simulink model "real_time_optimal_control"  (R2020b)
settings: Solver=ode4  StartTime=0.0  StopTime=30  FixedStep=h_plant  RelTol=1e-3
values from neighbouring files (symbols this model uses):
  A = [zeros(3) eye(3)   zeros(3) ... (first row only)    [run_drone_estimate.m]    (also in run_simulation.m = [0 1; 0 0])
  B = [zeros(3) zeros(3) ... (first row only)    [run_drone_estimate.m]    (also in run_simulation.m = [0; 1])
  C = [eye(3) zeros(3) zeros(3)]    [run_drone_estimate.m]    (also in run_simulation.m = [1 0])
  C_discrete = [1 0]    [run_simulation.m]
  D_discrete = zeros(3,6)    [run_drone_estimate.m]    (also in run_simulation.m = 0)
  G = [zeros(3) zeros(3) ... (first row only)    [run_drone_estimate.m]
  Gamma = [h^2/2; h]    [run_simulation.m]
  h = 0.1    [run_drone_estimate.m]    (also in run_simulation.m = 1)
  h_plant = (1e-3)    (= 0.001)    [run_drone_estimate.m]    (also in run_simulation.m)
  N = 20    [run_simulation.m]
  n = length(A)    [run_drone_estimate.m]    (also in run_simulation.m = length(Phi))
  Phi = [1 h; 0 1]    [run_simulation.m]
  Q = .1*eye(2*3)    [run_drone_estimate.m]
  Q0 = eye(n)    [run_simulation.m]
  Q1 = eye(n)    [run_simulation.m]
  Q2 = 1    [run_simulation.m]
  R = .1*eye(3)    [run_drone_estimate.m]
  reference = [am;g]    [run_drone_estimate.m]    (also in run_simulation.m = 0)
  sat_max = (10000)    (= 10000)    [run_drone_estimate.m]    (also in run_simulation.m = 10)
  sat_min = -(10000)    (= -10000)    [run_drone_estimate.m]    (also in run_simulation.m = -10)
  wind_final_value = 0    [run_drone_estimate.m]    (also in run_simulation.m)
  wind_initial_value = 0    [run_drone_estimate.m]    (also in run_simulation.m)
  wind_steptime = 5    [run_drone_estimate.m]    (also in run_simulation.m)
  x0 = zeros(n, 1)    [run_drone_estimate.m]    (also in run_simulation.m = zeros(2, 1))
undefined symbols (not defined in the file or in its folder): DiscIntNeverNeededParam, Discrete, K, K_non_optimal, Time
libraries: eeLuenbergerObserver x4, simulink x1, ctrlSharedLib x1
settings Model: Creator=Trevor  LastModifiedBy=lucas
settings SolverCC: AlgebraicLoopSolver=LineSearch  AutoInsertRateTranBlk=on
settings DataIOCC: LimitDataPoints=on  SaveFormat=Array
settings OptimizationCC: LifeSpan=inf
settings DebuggingCC: SFUnexpectedBacktrackingDiag=warning  SFNoUnconditionalDefaultTransitionDiag=warning  SFExecutionAtInitializationDiag=none  UnderSpecifiedDimensionMsg=warning  ArithmeticOperatorsInVariantConditions=warning
settings HardwareCC: ProdHWDeviceType=AMD->x86-64 (Windows64)
settings ModelReferenceCC: PropagateSignalLabelsOutOfModel=off
settings SFSimCC: SimUseLocalCustomCode=off  CustomCodeUndefinedFunction=UseInterfaceOnly
settings RTWCC: RTWUseLocalCustomCode=off
settings CodeAppCC: StateflowObjectComments=on
settings GRTTargetCC: TargetLangStandard=C89/C90 (ANSI)
settings ConfigComp: CovMetricSettings=dw  CovSaveCumulativeToWorkspaceVar=on  CovSaveSingleToWorkspaceVar=on  CovExternalEMLEnable=off

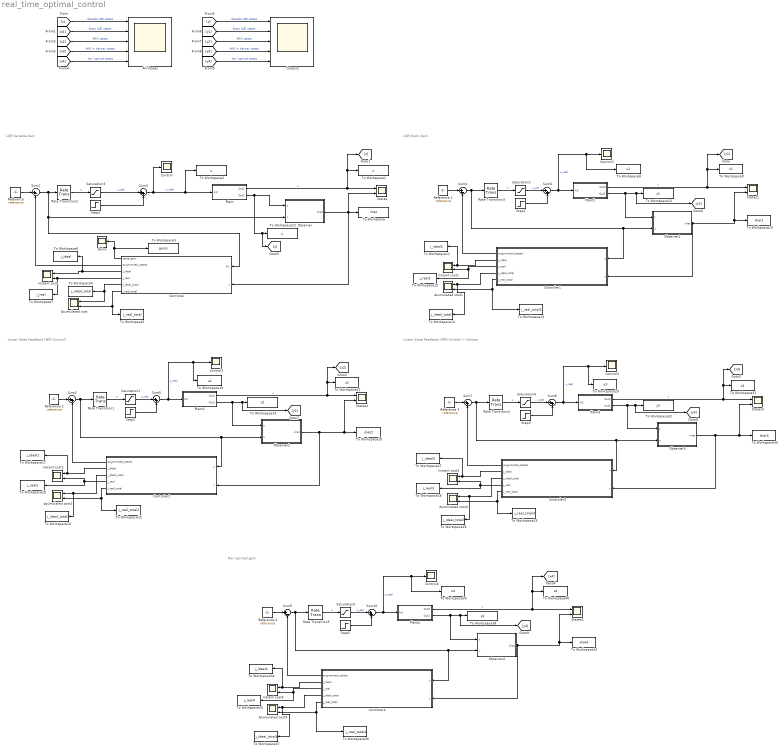
== system real_time_optimal_control ==
  note: LQR Static Gain
  note: LQR Variable Gain
  note: Linear State Feedback (MPC Control)
  note: Linear State Feedback (MPC Control) + Kalman
  note: Non optimal gain
  Acumulated cost{,1..4} (5 alike) : Scope  NumInputPorts=2
  All States : Scope  NumInputPorts=5
  Control{,1..4} (5 alike) : Scope
  Controler : Subsystem
  Controler1 : Subsystem
  Controler2 : Subsystem
  Controler3 : Subsystem
  Controler4 : Subsystem
  Gains : Scope
  Instant cost{,1..4} (5 alike) : Scope  NumInputPorts=2
  Observer : Subsystem
  Observer1 : Subsystem
  Observer2 : Subsystem
  Observer3 : Subsystem
  Observer4 : Subsystem
  Outputs : Scope  NumInputPorts=5
  Plant : Subsystem
  Plant1 : Subsystem
  Plant2 : Subsystem
  Plant3 : Subsystem
  Plant4 : Subsystem
  Rate Transition{1..5} (5 alike) : RateTransition  Integrity=off  OutPortSampleTimeMultiple=0.01  OutPortSampleTime=h_plant
  Reference : Constant  Value=reference  SampleTime=h
  Reference {1..4} (4 alike) : Constant  Value=reference  SampleTime=h
  Saturation{1..5} (5 alike) : Saturate  UpperLimit=sat_max  LowerLimit=sat_min
  States{,1..4} (5 alike) : Scope  NumInputPorts=2
  Step{1..5} (5 alike) : Step  Time=wind_steptime  Before=wind_initial_value  After=wind_final_value  SampleTime=h_plant
  Sum1 : Sum  Inputs=|+-
  Sum{2..3,5..8,10} (7 alike) : Sum  Inputs=|++
  Sum4 : Sum  Inputs=|+-
  Sum9 : Sum  Inputs=|+-
  To Workspace : ToWorkspace  VariableName=xhat  SaveFormat=Timeseries  SampleTime=-1
  To Workspace1 : ToWorkspace  VariableName=x  SaveFormat=Timeseries  SampleTime=-1
  To Workspace10 : ToWorkspace  VariableName=xhat1  SaveFormat=Timeseries  SampleTime=-1
  To Workspace11 : ToWorkspace  VariableName=j_ideal1  SaveFormat=Timeseries  SampleTime=-1
  To Workspace12 : ToWorkspace  VariableName=j_real1  SaveFormat=Timeseries  SampleTime=-1
  To Workspace13 : ToWorkspace  VariableName=j_real_total1  SaveFormat=Timeseries  SampleTime=-1
  To Workspace14 : ToWorkspace  VariableName=j_ideal_total1  SaveFormat=Timeseries  SampleTime=-1
  To Workspace15 : ToWorkspace  VariableName=j_real_total2  SaveFormat=Timeseries  SampleTime=-1
  To Workspace16 : ToWorkspace  VariableName=j_ideal_total2  SaveFormat=Timeseries  SampleTime=-1
  To Workspace17 : ToWorkspace  VariableName=j_ideal2  SaveFormat=Timeseries  SampleTime=-1
  To Workspace18 : ToWorkspace  VariableName=j_real2  SaveFormat=Timeseries  SampleTime=-1
  To Workspace19 : ToWorkspace  VariableName=u2  SaveFormat=Timeseries  SampleTime=-1
  To Workspace2 : ToWorkspace  VariableName=u  SaveFormat=Timeseries  SampleTime=-1
  To Workspace20 : ToWorkspace  VariableName=xhat2  SaveFormat=Timeseries  SampleTime=-1
  To Workspace21 : ToWorkspace  VariableName=x2  SaveFormat=Timeseries  SampleTime=-1
  To Workspace22 : ToWorkspace  VariableName=y  SaveFormat=Timeseries  SampleTime=-1
  To Workspace23 : ToWorkspace  VariableName=y1  SaveFormat=Timeseries  SampleTime=-1
  To Workspace24 : ToWorkspace  VariableName=y2  SaveFormat=Timeseries  SampleTime=-1
  To Workspace25 : ToWorkspace  VariableName=j_real_total3  SaveFormat=Timeseries  SampleTime=-1
  To Workspace26 : ToWorkspace  VariableName=j_ideal_total3  SaveFormat=Timeseries  SampleTime=-1
  To Workspace27 : ToWorkspace  VariableName=j_ideal3  SaveFormat=Timeseries  SampleTime=-1
  To Workspace28 : ToWorkspace  VariableName=j_real3  SaveFormat=Timeseries  SampleTime=-1
  To Workspace29 : ToWorkspace  VariableName=u3  SaveFormat=Timeseries  SampleTime=-1
  To Workspace3 : ToWorkspace  VariableName=gains  SaveFormat=Timeseries  SampleTime=-1
  To Workspace30 : ToWorkspace  VariableName=xhat3  SaveFormat=Timeseries  SampleTime=-1
  To Workspace31 : ToWorkspace  VariableName=x3  SaveFormat=Timeseries  SampleTime=-1
  To Workspace32 : ToWorkspace  VariableName=y3  SaveFormat=Timeseries  SampleTime=-1
  To Workspace33 : ToWorkspace  VariableName=xhat4  SaveFormat=Timeseries  SampleTime=-1
  To Workspace34 : ToWorkspace  VariableName=j_ideal4  SaveFormat=Timeseries  SampleTime=-1
  To Workspace35 : ToWorkspace  VariableName=j_real4  SaveFormat=Timeseries  SampleTime=-1
  To Workspace36 : ToWorkspace  VariableName=j_real_total4  SaveFormat=Timeseries  SampleTime=-1
  To Workspace37 : ToWorkspace  VariableName=j_ideal_total4  SaveFormat=Timeseries  SampleTime=-1
  To Workspace38 : ToWorkspace  VariableName=y4  SaveFormat=Timeseries  SampleTime=-1
  To Workspace39 : ToWorkspace  VariableName=u4  SaveFormat=Timeseries  SampleTime=-1
  To Workspace4 : ToWorkspace  VariableName=j_ideal_total  SaveFormat=Timeseries  SampleTime=-1
  To Workspace40 : ToWorkspace  VariableName=x4  SaveFormat=Timeseries  SampleTime=-1
  To Workspace5 : ToWorkspace  VariableName=j_real_total  SaveFormat=Timeseries  SampleTime=-1
  To Workspace6 : ToWorkspace  VariableName=j_ideal  SaveFormat=Timeseries  SampleTime=-1
  To Workspace7 : ToWorkspace  VariableName=j_real  SaveFormat=Timeseries  SampleTime=-1
  To Workspace8 : ToWorkspace  VariableName=u1  SaveFormat=Timeseries  SampleTime=-1
  To Workspace9 : ToWorkspace  VariableName=x1  SaveFormat=Timeseries  SampleTime=-1
  wires:
  Plant/2(Out1) -> [y], To Workspace22/1, Observer/1(y)
  Saturation3/1 -> Sum3/1  "u_sat"
  Sum3/1 -> Control/1, Plant/1(In2), To Workspace2/1  "u_real"
  Step4/1 -> Sum3/2
  Plant/1(Out2) -> [x], To Workspace1/1, States/1  "x"
  Reference/1 -> Sum1/1
  Rate Transition2/1 -> Saturation3/1  "u"
  Sum6/1 -> Plant1/1(In2), To Workspace8/1, Control1/1  "u_real"
  Step1/1 -> Sum6/2
  Plant1/1(Out2) -> [x1], To Workspace9/1, States1/1  "x"
  Reference 1/1 -> Sum4/1
  Sum4/1 -> Controler1/1(u), Observer1/2(u), Rate Transition3/1
  Observer1/1(xhat) -> Controler1/2(x), To Workspace10/1, States1/2
  Saturation1/1 -> Sum6/1  "u_sat"
  Plant1/2(Out1) -> Observer1/1(y), [y1], To Workspace23/1
  Rate Transition3/1 -> Saturation1/1  "u"
  Rate Transition1/1 -> Saturation2/1  "u"
  Saturation2/1 -> Sum5/1  "u_sat"
  Plant2/2(Out1) -> Observer2/1(y), [y2], To Workspace24/1
  Plant2/1(Out2) -> [x2], To Workspace21/1, States2/1  "x"
  Step2/1 -> Sum5/2
  Sum5/1 -> Plant2/1(In2), To Workspace19/1, Control2/1  "u_real"
  Sum2/1 -> Controler2/1(u), Observer2/2(u), Rate Transition1/1
  Reference 2/1 -> Sum2/1
  Sum1/1 -> Controler/1(In1), Observer/2(u), Rate Transition2/1
  Observer/1(xhat) -> To Workspace/1, Controler/2(x), States/2
  Controler/1(state_gain) -> To Workspace3/1, Gains/1
  Controler/2(augmented_states) -> Sum1/2
  Controler/3(j_ideal) -> To Workspace6/1, Instant cost/1
  Controler/4(j_real) -> To Workspace7/1, Instant cost/2
  Controler/5(j_ideal_total) -> Acumulated cost/1, To Workspace4/1
  Controler/6(j_real_total) -> To Workspace5/1, Acumulated cost/2
  Controler1/1(augmented_states) -> Sum4/2
  Controler1/2(j_ideal) -> To Workspace11/1, Instant cost1/1
  Controler1/3(j_real) -> To Workspace12/1, Instant cost1/2
  Controler1/4(j_ideal_total) -> To Workspace14/1, Acumulated cost1/1
  Controler1/5(j_real_total) -> To Workspace13/1, Acumulated cost1/2
  Controler2/3(j_ideal_total) -> To Workspace16/1, Acumulated cost2/1
  Controler2/5(j_real_total) -> To Workspace15/1, Acumulated cost2/2
  Controler2/2(j_ideal) -> To Workspace17/1, Instant cost2/1
  Observer2/1(xhat) -> Controler2/2(x), To Workspace20/1, States2/2
  Controler2/4(j_real) -> To Workspace18/1, Instant cost2/2
  Controler2/1(augmented_states) -> Sum2/2
  Controler3/4(j_real) -> To Workspace28/1, Instant cost3/2
  Sum8/1 -> Plant3/1(In2), To Workspace29/1, Control3/1  "u_real"
  Observer3/1(xhat) -> Controler3/2(x), To Workspace30/1, States3/2
  Step3/1 -> Sum8/2
  Plant3/2(Out1) -> Observer3/1(y), [y3], To Workspace32/1
  Saturation4/1 -> Sum8/1  "u_sat"
  Controler3/3(j_ideal_total) -> To Workspace26/1, Acumulated cost3/1
  Rate Transition4/1 -> Saturation4/1  "u"
  Sum7/1 -> Controler3/1(u), Observer3/2(u), Rate Transition4/1
  Reference 3/1 -> Sum7/1
  Plant3/1(Out2) -> [x3], To Workspace31/1, States3/1  "x"
  Controler3/2(j_ideal) -> To Workspace27/1, Instant cost3/1
  Controler3/5(j_real_total) -> To Workspace25/1, Acumulated cost3/2
  Controler3/1(augmented_states) -> Sum7/2
  [x] -> All States/1  "Variable LQR states"
  [x1] -> All States/2  "Static LQR states"
  [x2] -> All States/3  "MPC states"
  [x3] -> All States/4  "MPC + Kalman states"
  Reference 4/1 -> Sum9/1
  Controler4/5(j_real_total) -> To Workspace36/1, Acumulated cost4/2
  Controler4/1(augmented_states) -> Sum9/2
  Controler4/3(j_real) -> To Workspace35/1, Instant cost4/2
  Observer4/1(xhat) -> Controler4/2(x), To Workspace33/1, States4/2
  Controler4/4(j_ideal_total) -> To Workspace37/1, Acumulated cost4/1
  Step5/1 -> Sum10/2
  Rate Transition5/1 -> Saturation5/1  "u"
  Plant4/2(Out1) -> Observer4/1(y), [y4], To Workspace38/1
  Controler4/2(j_ideal) -> To Workspace34/1, Instant cost4/1
  Plant4/1(Out2) -> [x4], To Workspace40/1, States4/1  "x"
  Sum9/1 -> Controler4/1(u), Observer4/2(u), Rate Transition5/1
  Sum10/1 -> Plant4/1(In2), To Workspace39/1, Control4/1  "u_real"
  Saturation5/1 -> Sum10/1  "u_sat"
  [x4] -> All States/5  "Non optimal states"
  [y2] -> Outputs/3  "MPC states"
  [y3] -> Outputs/4  "MPC + Kalman states"
  [y] -> Outputs/1  "Variable LQR states"
  [y4] -> Outputs/5  "Non optimal states"
  [y1] -> Outputs/2  "Static LQR states"

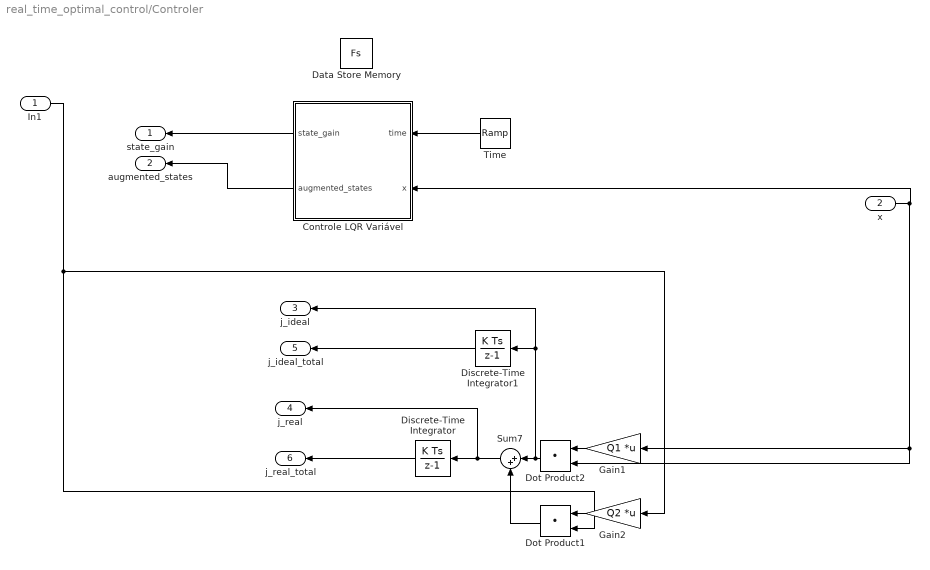
== system real_time_optimal_control/Controler ==
  In1 : Inport
  x : Inport  Port=2
  Controle LQR Variável : MATLAB Function  TreatAsAtomicUnit=on
  Data Store Memory : DataStoreMemory  DataStoreName=Fs  ReadBeforeWriteMsg=warning  WriteAfterWriteMsg=warning  WriteAfterReadMsg=warning  InitialValue=zeros(1,n,1,N)  VectorParams1D=off  ShowAdditionalParam=off  OutDataTypeStr=double
  Discrete-Time Integrator : DiscreteIntegrator  SampleTime=h  ICPrevOutput=DiscIntNeverNeededParam  ICPrevScaledInput=DiscIntNeverNeededParam
  Discrete-Time Integrator1 : DiscreteIntegrator  SampleTime=h  ICPrevOutput=DiscIntNeverNeededParam  ICPrevScaledInput=DiscIntNeverNeededParam
  Dot Product1 : DotProduct  InputSameDT=on  OutDataTypeStr=Inherit: Inherit via internal rule
  Dot Product2 : DotProduct  InputSameDT=on  OutDataTypeStr=Inherit: Inherit via internal rule
  Gain1 : Gain  Gain=Q1  Multiplication=Matrix(K*u)
  Gain2 : Gain  Gain=Q2  Multiplication=Matrix(K*u)
  Sum7 : Sum  Inputs=|++
  Time : simulink/Sources/Ramp  slope=h  start=0  InitialOutput=0
  state_gain : Outport
  augmented_states : Outport  Port=2
  j_ideal : Outport  Port=3
  j_real : Outport  Port=4
  j_ideal_total : Outport  Port=5
  j_real_total : Outport  Port=6
  wires:
  Gain1/1 -> Dot Product2/1
  In1/1 -> Dot Product1/2, Gain2/1
  Dot Product2/1 -> j_ideal/1, Discrete-Time Integrator1/1, Sum7/1
  Time/1 -> Controle LQR Variável/1(time)
  Controle LQR Variável/1(state_gain) -> state_gain/1
  Controle LQR Variável/2(augmented_states) -> augmented_states/1
  Gain2/1 -> Dot Product1/1
  x/1 -> Dot Product2/2, Gain1/1, Controle LQR Variável/2(x)
  Dot Product1/1 -> Sum7/2
  Sum7/1 -> j_real/1, Discrete-Time Integrator/1
  Discrete-Time Integrator1/1 -> j_ideal_total/1
  Discrete-Time Integrator/1 -> j_real_total/1

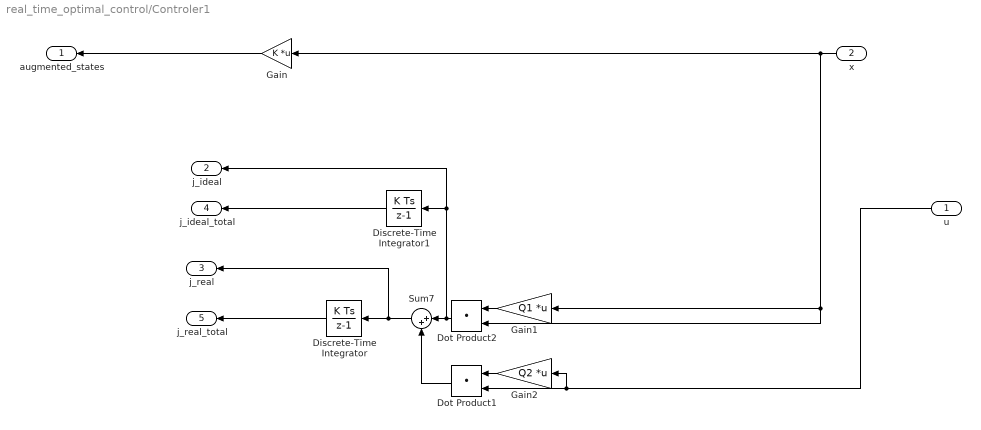
== system real_time_optimal_control/Controler1 ==
  u : Inport
  x : Inport  Port=2
  Discrete-Time Integrator : DiscreteIntegrator  SampleTime=h  ICPrevOutput=DiscIntNeverNeededParam  ICPrevScaledInput=DiscIntNeverNeededParam
  Discrete-Time Integrator1 : DiscreteIntegrator  SampleTime=h  ICPrevOutput=DiscIntNeverNeededParam  ICPrevScaledInput=DiscIntNeverNeededParam
  Dot Product1 : DotProduct  InputSameDT=on  OutDataTypeStr=Inherit: Inherit via internal rule
  Dot Product2 : DotProduct  InputSameDT=on  OutDataTypeStr=Inherit: Inherit via internal rule
  Gain : Gain  Gain=K  Multiplication=Matrix(K*u) (u vector)
  Gain1 : Gain  Gain=Q1  Multiplication=Matrix(K*u)
  Gain2 : Gain  Gain=Q2  Multiplication=Matrix(K*u)
  Sum7 : Sum  Inputs=|++
  augmented_states : Outport
  j_ideal : Outport  Port=2
  j_real : Outport  Port=3
  j_ideal_total : Outport  Port=4
  j_real_total : Outport  Port=5
  wires:
  Gain1/1 -> Dot Product2/1
  u/1 -> Gain2/1, Dot Product1/2
  Dot Product2/1 -> j_ideal/1, Discrete-Time Integrator1/1, Sum7/1
  Gain/1 -> augmented_states/1
  Gain2/1 -> Dot Product1/1
  x/1 -> Gain/1, Dot Product2/2, Gain1/1
  Dot Product1/1 -> Sum7/2
  Sum7/1 -> j_real/1, Discrete-Time Integrator/1
  Discrete-Time Integrator1/1 -> j_ideal_total/1
  Discrete-Time Integrator/1 -> j_real_total/1

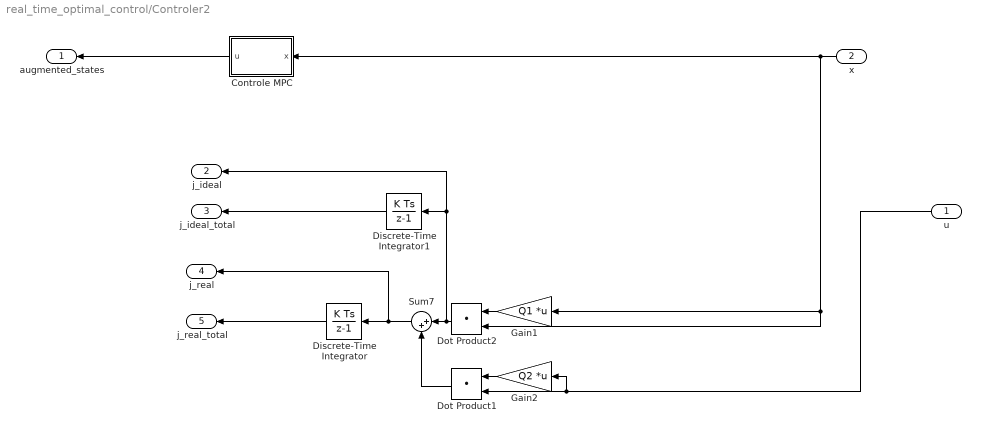
== system real_time_optimal_control/Controler2 ==
  u : Inport
  x : Inport  Port=2
  Controle MPC : MATLAB Function  TreatAsAtomicUnit=on
  Discrete-Time Integrator : DiscreteIntegrator  SampleTime=h  ICPrevOutput=DiscIntNeverNeededParam  ICPrevScaledInput=DiscIntNeverNeededParam
  Discrete-Time Integrator1 : DiscreteIntegrator  SampleTime=h  ICPrevOutput=DiscIntNeverNeededParam  ICPrevScaledInput=DiscIntNeverNeededParam
  Dot Product1 : DotProduct  InputSameDT=on  OutDataTypeStr=Inherit: Inherit via internal rule
  Dot Product2 : DotProduct  InputSameDT=on  OutDataTypeStr=Inherit: Inherit via internal rule
  Gain1 : Gain  Gain=Q1  Multiplication=Matrix(K*u)
  Gain2 : Gain  Gain=Q2  Multiplication=Matrix(K*u)
  Sum7 : Sum  Inputs=|++
  augmented_states : Outport
  j_ideal : Outport  Port=2
  j_ideal_total : Outport  Port=3
  j_real : Outport  Port=4
  j_real_total : Outport  Port=5
  wires:
  Gain1/1 -> Dot Product2/1
  u/1 -> Gain2/1, Dot Product1/2
  Dot Product2/1 -> j_ideal/1, Discrete-Time Integrator1/1, Sum7/1
  Controle MPC/1(u) -> augmented_states/1
  Gain2/1 -> Dot Product1/1
  x/1 -> Controle MPC/1(x), Dot Product2/2, Gain1/1
  Dot Product1/1 -> Sum7/2
  Sum7/1 -> j_real/1, Discrete-Time Integrator/1
  Discrete-Time Integrator1/1 -> j_ideal_total/1
  Discrete-Time Integrator/1 -> j_real_total/1

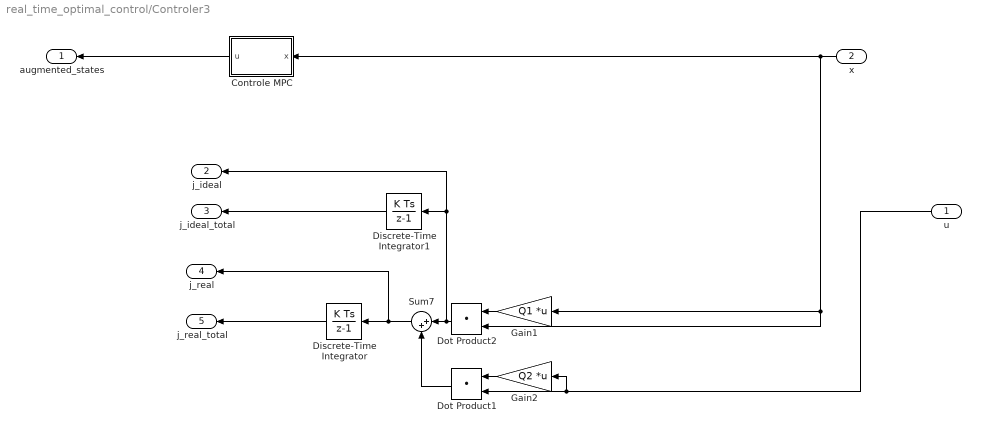
== system real_time_optimal_control/Controler3 ==
  u : Inport
  x : Inport  Port=2
  Controle MPC : MATLAB Function  TreatAsAtomicUnit=on
  Discrete-Time Integrator : DiscreteIntegrator  SampleTime=h  ICPrevOutput=DiscIntNeverNeededParam  ICPrevScaledInput=DiscIntNeverNeededParam
  Discrete-Time Integrator1 : DiscreteIntegrator  SampleTime=h  ICPrevOutput=DiscIntNeverNeededParam  ICPrevScaledInput=DiscIntNeverNeededParam
  Dot Product1 : DotProduct  InputSameDT=on  OutDataTypeStr=Inherit: Inherit via internal rule
  Dot Product2 : DotProduct  InputSameDT=on  OutDataTypeStr=Inherit: Inherit via internal rule
  Gain1 : Gain  Gain=Q1  Multiplication=Matrix(K*u)
  Gain2 : Gain  Gain=Q2  Multiplication=Matrix(K*u)
  Sum7 : Sum  Inputs=|++
  augmented_states : Outport
  j_ideal : Outport  Port=2
  j_ideal_total : Outport  Port=3
  j_real : Outport  Port=4
  j_real_total : Outport  Port=5
  wires:
  Gain1/1 -> Dot Product2/1
  u/1 -> Gain2/1, Dot Product1/2
  Dot Product2/1 -> j_ideal/1, Discrete-Time Integrator1/1, Sum7/1
  Controle MPC/1(u) -> augmented_states/1
  Gain2/1 -> Dot Product1/1
  x/1 -> Controle MPC/1(x), Dot Product2/2, Gain1/1
  Dot Product1/1 -> Sum7/2
  Sum7/1 -> j_real/1, Discrete-Time Integrator/1
  Discrete-Time Integrator1/1 -> j_ideal_total/1
  Discrete-Time Integrator/1 -> j_real_total/1

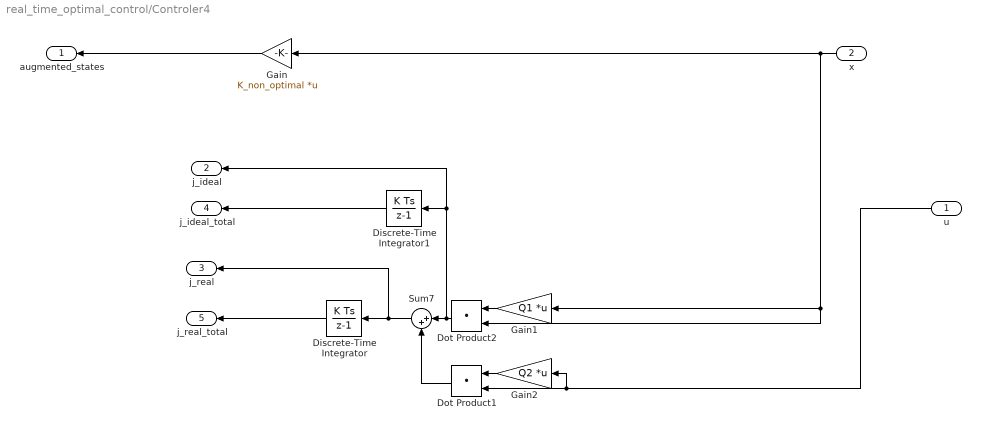
== system real_time_optimal_control/Controler4 ==
  u : Inport
  x : Inport  Port=2
  Discrete-Time Integrator : DiscreteIntegrator  SampleTime=h  ICPrevOutput=DiscIntNeverNeededParam  ICPrevScaledInput=DiscIntNeverNeededParam
  Discrete-Time Integrator1 : DiscreteIntegrator  SampleTime=h  ICPrevOutput=DiscIntNeverNeededParam  ICPrevScaledInput=DiscIntNeverNeededParam
  Dot Product1 : DotProduct  InputSameDT=on  OutDataTypeStr=Inherit: Inherit via internal rule
  Dot Product2 : DotProduct  InputSameDT=on  OutDataTypeStr=Inherit: Inherit via internal rule
  Gain : Gain  Gain=K_non_optimal  Multiplication=Matrix(K*u) (u vector)
  Gain1 : Gain  Gain=Q1  Multiplication=Matrix(K*u)
  Gain2 : Gain  Gain=Q2  Multiplication=Matrix(K*u)
  Sum7 : Sum  Inputs=|++
  augmented_states : Outport
  j_ideal : Outport  Port=2
  j_real : Outport  Port=3
  j_ideal_total : Outport  Port=4
  j_real_total : Outport  Port=5
  wires:
  Gain1/1 -> Dot Product2/1
  u/1 -> Gain2/1, Dot Product1/2
  Dot Product2/1 -> j_ideal/1, Discrete-Time Integrator1/1, Sum7/1
  Gain/1 -> augmented_states/1
  Gain2/1 -> Dot Product1/1
  x/1 -> Gain/1, Dot Product2/2, Gain1/1
  Dot Product1/1 -> Sum7/2
  Sum7/1 -> j_real/1, Discrete-Time Integrator/1
  Discrete-Time Integrator1/1 -> j_ideal_total/1
  Discrete-Time Integrator/1 -> j_real_total/1

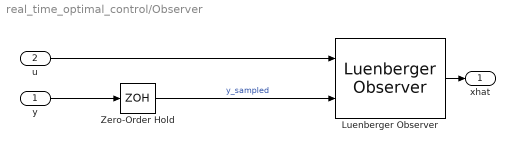
== system real_time_optimal_control/Observer ==
  y : Inport
  u : Inport  Port=2
  Luenberger Observer : eeLuenbergerObserver/Luenberger Observer  StateSpaceType=Discrete-time  Ad=Phi  Bd=Gamma  Cd=C_discrete  Dd=D_discrete  A=1  B=1  C=1  D=1  ObserverDesign=Desired eigenvalues  Ld=1  DesiredEigenvalues=observer_eig  x0=x0_observer  Tsd=0.1  Ts=h
      settings: SourceProductBaseCode=PS
  Zero-Order Hold : ZeroOrderHold  SampleTime=h
  xhat : Outport
  wires:
  Zero-Order Hold/1 -> Luenberger Observer/2  "y_sampled"
  Luenberger Observer/1 -> xhat/1
  y/1 -> Zero-Order Hold/1
  u/1 -> Luenberger Observer/1

== system real_time_optimal_control/Observer1 ==
  y : Inport
  u : Inport  Port=2
  Luenberger Observer : eeLuenbergerObserver/Luenberger Observer  StateSpaceType=Discrete-time  Ad=Phi  Bd=Gamma  Cd=C_discrete  Dd=D_discrete  A=1  B=1  C=1  D=1  ObserverDesign=Desired eigenvalues  Ld=observer_gain  DesiredEigenvalues=observer_eig  x0=x0_observer  Tsd=0.1  Ts=h
      settings: SourceProductBaseCode=PS
  Zero-Order Hold : ZeroOrderHold  SampleTime=h
  xhat : Outport
  wires:
  Zero-Order Hold/1 -> Luenberger Observer/2  "y_sampled"
  Luenberger Observer/1 -> xhat/1
  y/1 -> Zero-Order Hold/1
  u/1 -> Luenberger Observer/1

== system real_time_optimal_control/Observer2 ==
  y : Inport
  u : Inport  Port=2
  Luenberger Observer : eeLuenbergerObserver/Luenberger Observer  StateSpaceType=Discrete-time  Ad=Phi  Bd=Gamma  Cd=C_discrete  Dd=D_discrete  A=1  B=1  C=1  D=1  ObserverDesign=Desired eigenvalues  Ld=1  DesiredEigenvalues=observer_eig  x0=x0_observer  Tsd=0.1  Ts=h
      settings: SourceProductBaseCode=PS
  Zero-Order Hold : ZeroOrderHold  SampleTime=h
  xhat : Outport
  wires:
  Zero-Order Hold/1 -> Luenberger Observer/2  "y_sampled"
  Luenberger Observer/1 -> xhat/1
  y/1 -> Zero-Order Hold/1
  u/1 -> Luenberger Observer/1

== system real_time_optimal_control/Observer3 ==
  y : Inport
  u : Inport  Port=2
  Kalman Filter1 : ctrlSharedLib/Kalman Filter  TimeDomain=Discrete-Time  UseCurrentEstimator=on  ModelSource=Individual A, B, C, D matrices  ModelSourceVariable=ss(0.95,1,1,0,1)  A=Phi  B=Gamma  C=C_discrete  D=D_discrete  NumberOfStates=1  NumberOfInputs=1  NumberOfOutputs=1  InitialEstimateSource=Dialog  X0=zeros(n, 1)  P0=eye(n)  UseK=off  UseGH=on  NumberOfProcessNoiseInputs=1  G=G  TimeInvariantG=on  H=0  TimeInvariantH=on  Q=Q  TimeInvariantQ=on  R=R  TimeInvariantR=on  N=0  TimeInvariantN=on  AddInputPort=on  AddEnablePort=off  OutputEstimatedY=off  OutputP=off  Ts=-1
  Zero-Order Hold : ZeroOrderHold  SampleTime=h
  xhat : Outport
  wires:
  Zero-Order Hold/1 -> Kalman Filter1/2  "y_sampled"
  y/1 -> Zero-Order Hold/1
  u/1 -> Kalman Filter1/1
  Kalman Filter1/1 -> xhat/1

== system real_time_optimal_control/Observer4 ==
  y : Inport
  u : Inport  Port=2
  Luenberger Observer : eeLuenbergerObserver/Luenberger Observer  StateSpaceType=Discrete-time  Ad=Phi  Bd=Gamma  Cd=C_discrete  Dd=D_discrete  A=1  B=1  C=1  D=1  ObserverDesign=Desired eigenvalues  Ld=observer_gain  DesiredEigenvalues=observer_eig  x0=x0_observer  Tsd=0.1  Ts=h
      settings: SourceProductBaseCode=PS
  Zero-Order Hold : ZeroOrderHold  SampleTime=h
  xhat : Outport
  wires:
  Zero-Order Hold/1 -> Luenberger Observer/2  "y_sampled"
  Luenberger Observer/1 -> xhat/1
  y/1 -> Zero-Order Hold/1
  u/1 -> Luenberger Observer/1

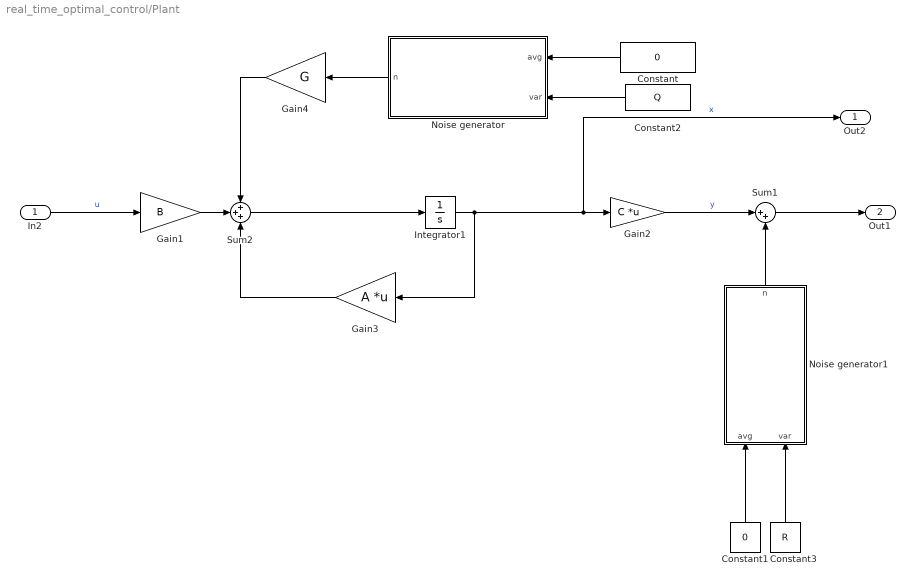
== system real_time_optimal_control/Plant ==
  In2 : Inport
  Constant : Constant  Value=0  VectorParams1D=off
  Constant1 : Constant  Value=0
  Constant2 : Constant  Value=Q
  Constant3 : Constant  Value=R
  Gain1 : Gain  Gain=B
  Gain2 : Gain  Gain=C  Multiplication=Matrix(K*u) (u vector)
  Gain3 : Gain  Gain=A  Multiplication=Matrix(K*u) (u vector)
  Gain4 : Gain  Gain=G
  Integrator1 : Integrator  InitialCondition=x0
  Noise generator : MATLAB Function  TreatAsAtomicUnit=on
  Noise generator1 : MATLAB Function  TreatAsAtomicUnit=on
  Sum1 : Sum  Inputs=|++
  Sum2 : Sum  Inputs=+++
  Out2 : Outport
  Out1 : Outport  Port=2
  wires:
  Gain2/1 -> Sum1/1  "y"
  Constant1/1 -> Noise generator1/1(avg)
  Sum1/1 -> Out1/1
  Noise generator1/1(n) -> Sum1/2
  Gain4/1 -> Sum2/1
  Gain3/1 -> Sum2/3
  Gain1/1 -> Sum2/2
  Constant2/1 -> Noise generator/2(var)
  Constant/1 -> Noise generator/1(avg)
  Integrator1/1 -> Gain3/1, Out2/1, Gain2/1  "x"
  In2/1 -> Gain1/1  "u"
  Constant3/1 -> Noise generator1/2(var)
  Noise generator/1(n) -> Gain4/1
  Sum2/1 -> Integrator1/1

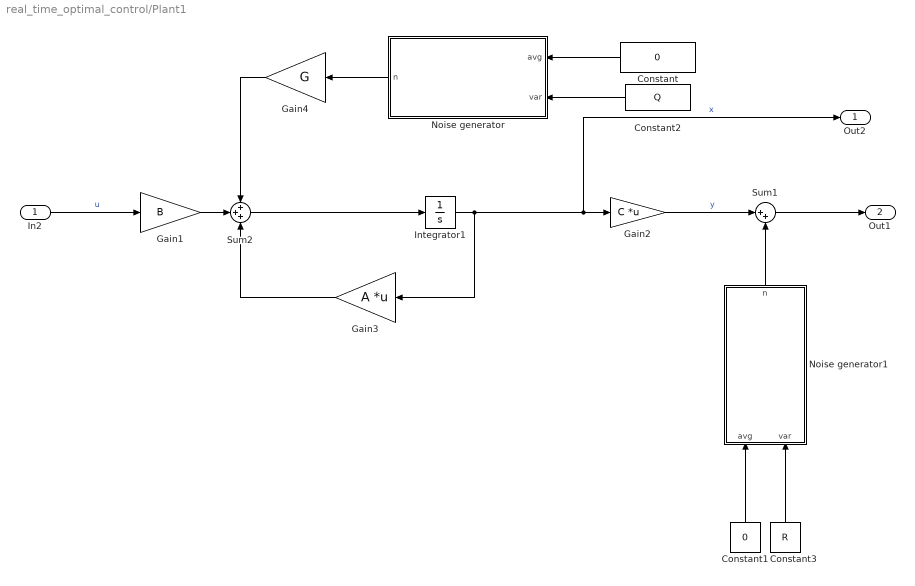
== system real_time_optimal_control/Plant1 ==
  In2 : Inport
  Constant : Constant  Value=0  VectorParams1D=off
  Constant1 : Constant  Value=0
  Constant2 : Constant  Value=Q
  Constant3 : Constant  Value=R
  Gain1 : Gain  Gain=B
  Gain2 : Gain  Gain=C  Multiplication=Matrix(K*u) (u vector)
  Gain3 : Gain  Gain=A  Multiplication=Matrix(K*u) (u vector)
  Gain4 : Gain  Gain=G
  Integrator1 : Integrator  InitialCondition=x0
  Noise generator : MATLAB Function  TreatAsAtomicUnit=on
  Noise generator1 : MATLAB Function  TreatAsAtomicUnit=on
  Sum1 : Sum  Inputs=|++
  Sum2 : Sum  Inputs=+++
  Out2 : Outport
  Out1 : Outport  Port=2
  wires:
  Gain2/1 -> Sum1/1  "y"
  Constant1/1 -> Noise generator1/1(avg)
  Sum1/1 -> Out1/1
  Noise generator1/1(n) -> Sum1/2
  Gain4/1 -> Sum2/1
  Gain3/1 -> Sum2/3
  Gain1/1 -> Sum2/2
  Constant2/1 -> Noise generator/2(var)
  Constant/1 -> Noise generator/1(avg)
  Integrator1/1 -> Gain3/1, Out2/1, Gain2/1  "x"
  In2/1 -> Gain1/1  "u"
  Constant3/1 -> Noise generator1/2(var)
  Noise generator/1(n) -> Gain4/1
  Sum2/1 -> Integrator1/1

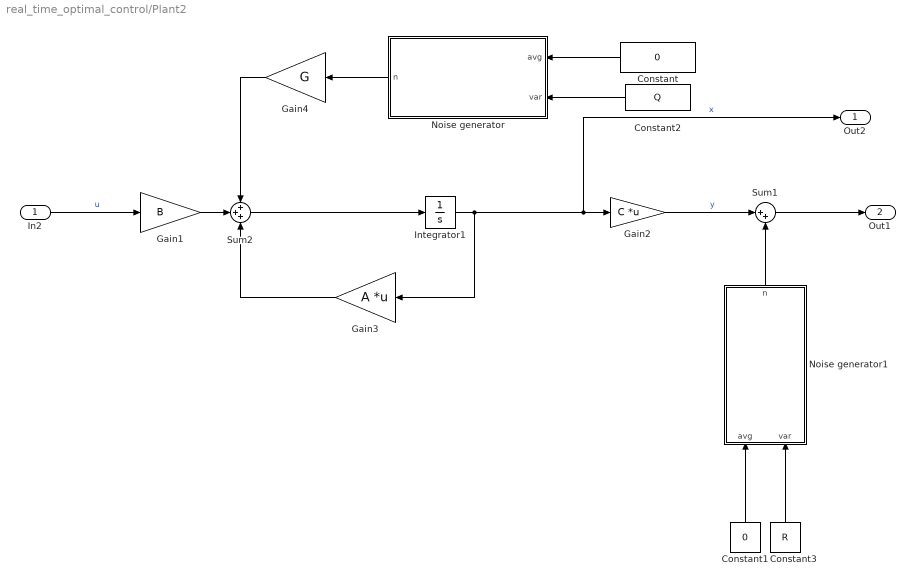
== system real_time_optimal_control/Plant2 ==
  In2 : Inport
  Constant : Constant  Value=0  VectorParams1D=off
  Constant1 : Constant  Value=0
  Constant2 : Constant  Value=Q
  Constant3 : Constant  Value=R
  Gain1 : Gain  Gain=B
  Gain2 : Gain  Gain=C  Multiplication=Matrix(K*u) (u vector)
  Gain3 : Gain  Gain=A  Multiplication=Matrix(K*u) (u vector)
  Gain4 : Gain  Gain=G
  Integrator1 : Integrator  InitialCondition=x0
  Noise generator : MATLAB Function  TreatAsAtomicUnit=on
  Noise generator1 : MATLAB Function  TreatAsAtomicUnit=on
  Sum1 : Sum  Inputs=|++
  Sum2 : Sum  Inputs=+++
  Out2 : Outport
  Out1 : Outport  Port=2
  wires:
  Gain2/1 -> Sum1/1  "y"
  Constant1/1 -> Noise generator1/1(avg)
  Sum1/1 -> Out1/1
  Noise generator1/1(n) -> Sum1/2
  Gain4/1 -> Sum2/1
  Gain3/1 -> Sum2/3
  Gain1/1 -> Sum2/2
  Constant2/1 -> Noise generator/2(var)
  Constant/1 -> Noise generator/1(avg)
  Integrator1/1 -> Gain3/1, Out2/1, Gain2/1  "x"
  In2/1 -> Gain1/1  "u"
  Constant3/1 -> Noise generator1/2(var)
  Noise generator/1(n) -> Gain4/1
  Sum2/1 -> Integrator1/1

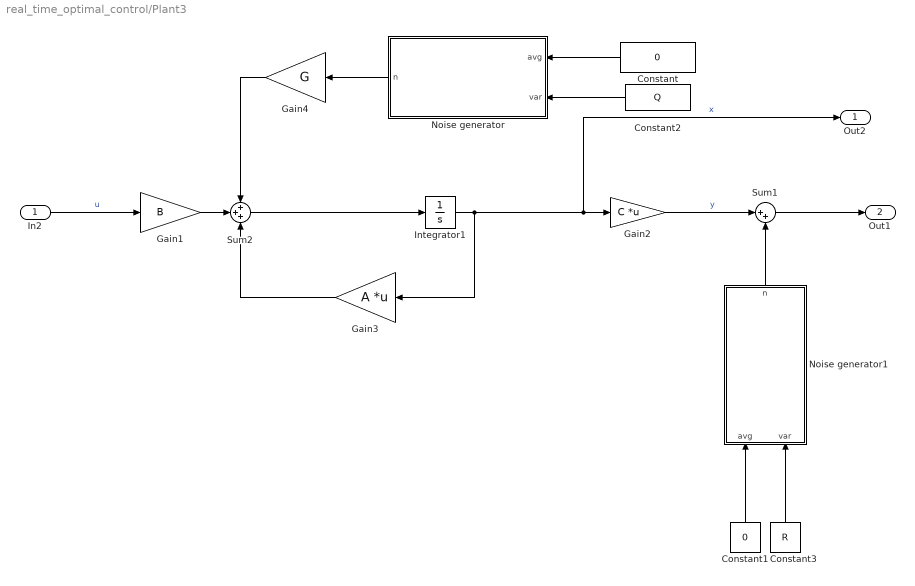
== system real_time_optimal_control/Plant3 ==
  In2 : Inport
  Constant : Constant  Value=0  VectorParams1D=off
  Constant1 : Constant  Value=0
  Constant2 : Constant  Value=Q
  Constant3 : Constant  Value=R
  Gain1 : Gain  Gain=B
  Gain2 : Gain  Gain=C  Multiplication=Matrix(K*u) (u vector)
  Gain3 : Gain  Gain=A  Multiplication=Matrix(K*u) (u vector)
  Gain4 : Gain  Gain=G
  Integrator1 : Integrator  InitialCondition=x0
  Noise generator : MATLAB Function  TreatAsAtomicUnit=on
  Noise generator1 : MATLAB Function  TreatAsAtomicUnit=on
  Sum1 : Sum  Inputs=|++
  Sum2 : Sum  Inputs=+++
  Out2 : Outport
  Out1 : Outport  Port=2
  wires:
  Sum2/1 -> Integrator1/1
  Gain2/1 -> Sum1/1  "y"
  Sum1/1 -> Out1/1
  In2/1 -> Gain1/1  "u"
  Integrator1/1 -> Gain3/1, Out2/1, Gain2/1  "x"
  Gain1/1 -> Sum2/2
  Gain3/1 -> Sum2/3
  Noise generator/1(n) -> Gain4/1
  Gain4/1 -> Sum2/1
  Constant/1 -> Noise generator/1(avg)
  Constant1/1 -> Noise generator1/1(avg)
  Constant3/1 -> Noise generator1/2(var)
  Noise generator1/1(n) -> Sum1/2
  Constant2/1 -> Noise generator/2(var)

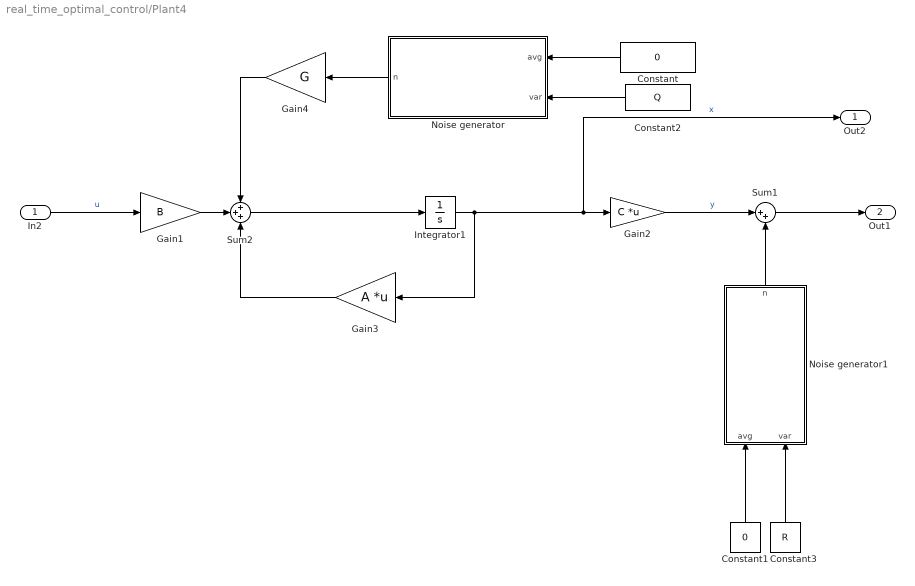
== system real_time_optimal_control/Plant4 ==
  In2 : Inport
  Constant : Constant  Value=0  VectorParams1D=off
  Constant1 : Constant  Value=0
  Constant2 : Constant  Value=Q
  Constant3 : Constant  Value=R
  Gain1 : Gain  Gain=B
  Gain2 : Gain  Gain=C  Multiplication=Matrix(K*u) (u vector)
  Gain3 : Gain  Gain=A  Multiplication=Matrix(K*u) (u vector)
  Gain4 : Gain  Gain=G
  Integrator1 : Integrator  InitialCondition=x0
  Noise generator : MATLAB Function  TreatAsAtomicUnit=on
  Noise generator1 : MATLAB Function  TreatAsAtomicUnit=on
  Sum1 : Sum  Inputs=|++
  Sum2 : Sum  Inputs=+++
  Out2 : Outport
  Out1 : Outport  Port=2
  wires:
  Gain2/1 -> Sum1/1  "y"
  Constant1/1 -> Noise generator1/1(avg)
  Sum1/1 -> Out1/1
  Noise generator1/1(n) -> Sum1/2
  Gain4/1 -> Sum2/1
  Gain3/1 -> Sum2/3
  Gain1/1 -> Sum2/2
  Constant2/1 -> Noise generator/2(var)
  Constant/1 -> Noise generator/1(avg)
  Integrator1/1 -> Gain3/1, Out2/1, Gain2/1  "x"
  In2/1 -> Gain1/1  "u"
  Constant3/1 -> Noise generator1/2(var)
  Noise generator/1(n) -> Gain4/1
  Sum2/1 -> Integrator1/1

== matlab function real_time_optimal_control/Plant/Noise generator ==
  data: avg input; n output; var input
function n = generate_gaussian_noise(avg, var)
n = avg + var.*randn(length(var), 1);

== matlab function real_time_optimal_control/Plant/Noise generator1 ==
  data: avg input; n output; var input
function n = generate_gaussian_noise(avg, var)
n = avg + var.*randn(length(var), 1);

== matlab function real_time_optimal_control/Plant1/Noise generator ==
  data: avg input; n output; var input
function n = generate_gaussian_noise(avg, var)
n = avg + var.*randn(length(var), 1);

== matlab function real_time_optimal_control/Plant1/Noise generator1 ==
  data: avg input; n output; var input
function n = generate_gaussian_noise(avg, var)
n = avg + var.*randn(length(var), 1);

== matlab function real_time_optimal_control/Plant2/Noise generator ==
  data: avg input; n output; var input
function n = generate_gaussian_noise(avg, var)
n = avg + var.*randn(length(var), 1);

== matlab function real_time_optimal_control/Plant2/Noise generator1 ==
  data: avg input; n output; var input
function n = generate_gaussian_noise(avg, var)
n = avg + var.*randn(length(var), 1);

== matlab function real_time_optimal_control/Plant4/Noise generator ==
  data: avg input; n output; var input
function n = generate_gaussian_noise(avg, var)
n = avg + var.*randn(length(var), 1);

== matlab function real_time_optimal_control/Plant4/Noise generator1 ==
  data: avg input; n output; var input
function n = generate_gaussian_noise(avg, var)
n = avg + var.*randn(length(var), 1);

== matlab function real_time_optimal_control/Controler2/Controle MPC ==
  settings: updateMethod=DISCRETE  sampleTime=h
  data: Q1 parameter; Q2 parameter; Q0 parameter; n parameter; Phi parameter; Gamma parameter; x input; N parameter; u output
function u  = mpc(Q1,Q2,Q0,n,Phi,Gamma,x,N)
%#codegen

tStart = tic;

coder.extrinsic('quadprog');

U = zeros(N,1);
Gain = zeros(2,1);
fval = 0;
z = zeros(N,1);

M0 = [Phi];
coder.varsize("Mu");
Mu = [Gamma, zeros(size(Gamma,1), N-1)];
Mu_aux = Mu;
Qtil =  kron(eye((N-1)*(n-1)), Q1);
Rbar = kron(eye(N*size(Gamma,2)), Q2);
Qbar = blkdiag(Qtil, Q0);
for i = 1:N-1
    M0 = [M0; Phi^(i+1)];
end
for i = 1:N-1
    Mu_aux = [Mu_aux(1)*Gamma, Mu_aux(:,1:length(Mu_aux)-1)];
    Mu = [Mu; Mu_aux];
end
Qxo = Q1 + M0'*Qbar*M0;
Qu = 2*Mu'*Qbar*Mu + Rbar;
Qxu = 2*M0'*Qbar*Mu;


[U , fval] = quadprog(2*Qu, 2*Qxu'*x);%, G_teste, W_teste + S_teste*x);
u = U(1,:);

tEnd = toc(tStart);

== matlab function real_time_optimal_control/Controler3/Controle MPC ==
  settings: updateMethod=DISCRETE  sampleTime=h
  data: Q1 parameter; Q2 parameter; Q0 parameter; n parameter; Phi parameter; Gamma parameter; x input; N parameter; u output
function u  = mpc(Q1,Q2,Q0,n,Phi,Gamma,x,N)
%#codegen

tStart = tic;

coder.extrinsic('quadprog');

U = zeros(N,1);
Gain = zeros(2,1);
fval = 0;
z = zeros(N,1);

M0 = [Phi];
coder.varsize("Mu");
Mu = [Gamma, zeros(size(Gamma,1), N-1)];
Mu_aux = Mu;
Qtil =  kron(eye((N-1)*(n-1)), Q1);
Rbar = kron(eye(N*size(Gamma,2)), Q2);
Qbar = blkdiag(Qtil, Q0);
for i = 1:N-1
    M0 = [M0; Phi^(i+1)];
end
for i = 1:N-1
    Mu_aux = [Mu_aux(1)*Gamma, Mu_aux(:,1:length(Mu_aux)-1)];
    Mu = [Mu; Mu_aux];
end
Qxo = Q1 + M0'*Qbar*M0;
Qu = 2*Mu'*Qbar*Mu + Rbar;
Qxu = 2*M0'*Qbar*Mu;


[U , fval] = quadprog(2*Qu, 2*Qxu'*x);%, G_teste, W_teste + S_teste*x);
u = U(1,:);

tEnd = toc(tStart);

== matlab function real_time_optimal_control/Plant3/Noise generator ==
  data: avg input; n output; var input
function n = generate_gaussian_noise(avg, var)
n = avg + var.*randn(length(var), 1);

== matlab function real_time_optimal_control/Plant3/Noise generator1 ==
  data: avg input; n output; var input
function n = generate_gaussian_noise(avg, var)
n = avg + var.*randn(length(var), 1);

== matlab function real_time_optimal_control/Controler/Controle LQR Variável ==
  settings: updateMethod=DISCRETE  sampleTime=h
  data: state_gain output; augmented_states output; time input; x input; h parameter; n parameter; N parameter; Q0 parameter; Q1 parameter; Phi parameter; Gamma parameter; Q2 parameter; Fs data_store_memory
function [state_gain, augmented_states]  = LQR(time, x, h, n, N, Q0, Q1, Phi, Gamma, Q2)
    global Fs; %datastores
    idx = 1 + mod(floor(time/h),N);
    if (idx == 1)
        S = zeros(n,n,1,N+1);
        S(:,:,1,N+1) = Q0;
        for j=(N):-1:1
            first_val = Q1;
            second_val = (Phi' * S(:,:,1,j+1) * Phi);
            third_val = (Phi' * S(:,:,1,j+1) * Gamma)*(((Gamma' * S(:,:,1,j+1) * Gamma) + Q2)\(Gamma' * S(:,:,1,j+1) * Phi));
            S(:,:,1,j) = first_val + second_val - third_val;
            Fs(:,:,1,j) = ((Gamma' * S(:,:,1,j+1) * Gamma) + Q2)\(Gamma' * S(:,:,1,j+1) * Phi);
        end
    end
    state_gain = Fs(:,:,1,idx);
    augmented_states = state_gain*x;
